simulink model "Hybrid_final_project_computer"  (R2022a)
settings: Solver=FixedStepAuto  StartTime=0.0  StopTime=25.0  RelTol=1e-3
model workspace (MAT data in the model file):
  Constant_a = Simulink.Parameter
  Constant_a.Value = [0  0.3  0.4  0.3; 0.3  0  0.5  0; 0.4  0.5  0  0.3; 0.3  0  0.3  0]
  Constant_a.DataType = 'auto'
  Constant_a.Complexity = 'real'
  Constant_a.Dimensions = [4 4]
  Constant_b = Simulink.Parameter
  Constant_b.Value = [0.3; 0.2; 0.5; 0.4]
  Constant_b.DataType = 'auto'
  Constant_b.Complexity = 'real'
  Constant_b.Dimensions = [4 1]
  Initial_Room_Temps = Simulink.Parameter
  Initial_Room_Temps.Value = [16.5; 16.5; 16.5; 16.5]
  Initial_Room_Temps.DataType = 'auto'
  Initial_Room_Temps.Complexity = 'real'
  Initial_Room_Temps.Dimensions = [4 1]
  constant_c = Simulink.Parameter
  constant_c.Value = [9; 7; 11; 7]
  constant_c.DataType = 'auto'
  constant_c.Complexity = 'real'
  constant_c.Dimensions = [4 1]
  dif_temps = Simulink.Parameter
  dif_temps.Value = [1; 1; 1; 1]
  dif_temps.DataType = 'auto'
  dif_temps.Complexity = 'real'
  dif_temps.Dimensions = [4 1]
  get_temps = Simulink.Parameter
  get_temps.Value = [17; 16; 16; 17]
  get_temps.DataType = 'auto'
  get_temps.Complexity = 'real'
  get_temps.Dimensions = [4 1]
  initial_placement = Simulink.Parameter
  initial_placement.Value = [0; 1; 1; 0]
  initial_placement.DataType = 'auto'
  initial_placement.Complexity = 'real'
  initial_placement.Dimensions = [4 1]
  off_temps = Simulink.Parameter
  off_temps.Value = [20; 20; 20; 20]
  off_temps.DataType = 'auto'
  off_temps.Complexity = 'real'
  off_temps.Dimensions = [4 1]
  on_temps = Simulink.Parameter
  on_temps.Value = [19; 19; 19; 19]
  on_temps.DataType = 'auto'
  on_temps.Complexity = 'real'
  on_temps.Dimensions = [4 1]
settings Model: Creator=jamieshatsky  LastModifiedBy=jamieshatsky
settings DebuggingCC: UnderSpecifiedDimensionMsg=warning

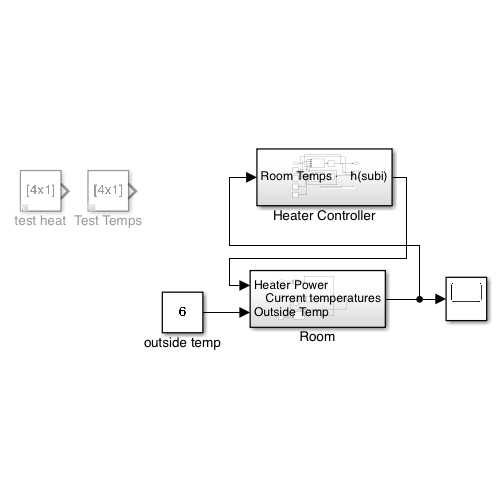
[thumbnail: Simulink's stored preview of the top-level diagram]
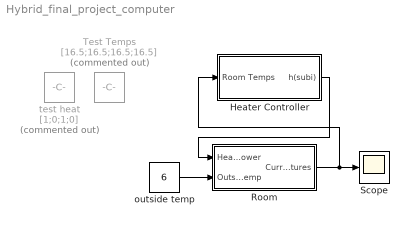
== system Hybrid_final_project_computer ==
  Heater Controller : Subsystem
  Room : Subsystem
  Scope : Scope
  Test Temps : Constant  Commented=on  Value=[16.5;16.5;16.5;16.5]
  outside temp : Constant  Value=6
  test heat : Constant  Commented=on  Value=[1;0;1;0]
  wires:
  outside temp/1 -> Room/2(Outside Temp)
  Room/1(Current temperatures) -> Heater Controller/1(Room Temps), Scope/1
  Heater Controller/1(h(subi)) -> Room/1(Heater Power)

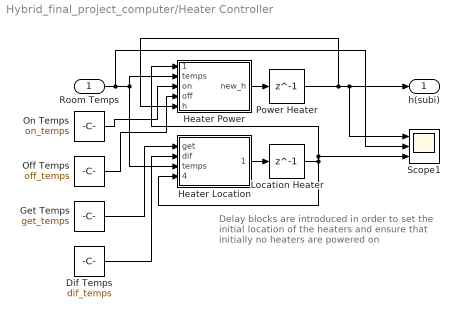
== system Hybrid_final_project_computer/Heater Controller ==
  note: Delay blocks are introduced in order to set the initial location of the heaters
      | and ensure that initially no heaters are powered on
  Room Temps : Inport
  Dif Temps : Constant  Value=dif_temps
  Get Temps : Constant  Value=get_temps
  Heater Location : MATLAB Function  TreatAsAtomicUnit=on
  Heater Power : MATLAB Function  TreatAsAtomicUnit=on
  Location Heater : Delay  DelayLength=1  InitialCondition=initial_placement
  Off Temps : Constant  Value=off_temps
  On Temps : Constant  Value=on_temps
  Power Heater : Delay  DelayLength=1  InitialCondition=[0;0;0;0]
  Scope1 : Scope  NumInputPorts=3
  h(subi) : Outport
  wires:
  Heater Location/1(new_location) -> Location Heater/1
  Room Temps/1 -> Scope1/2, Heater Location/3(temps), Heater Power/2(temps)
  Location Heater/1 -> Heater Power/1(location), Scope1/3, Heater Location/4(location)
  On Temps/1 -> Heater Power/3(on)
  Off Temps/1 -> Heater Power/4(off)
  Get Temps/1 -> Heater Location/1(get)
  Dif Temps/1 -> Heater Location/2(dif)
  Heater Power/1(new_h) -> Power Heater/1
  Power Heater/1 -> Scope1/1, h(subi)/1, Heater Power/5(h)

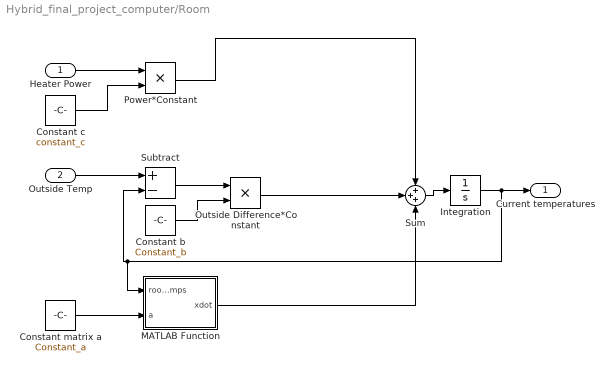
== system Hybrid_final_project_computer/Room ==
  Heater Power : Inport  PortDimensions=4
  Outside Temp : Inport  Port=2
  Constant b : Constant  Value=Constant_b
  Constant c : Constant  Value=constant_c
  Constant matrix a : Constant  Value=Constant_a  VectorParams1D=off
  Integration : Integrator  InitialCondition=Initial_Room_Temps
  MATLAB Function : MATLAB Function  TreatAsAtomicUnit=on
  Outside Difference*Constant : Product
  Power*Constant : Product
  Subtract : Sum  Inputs=+-
  Sum : Sum  Inputs=+++
  Current temperatures : Outport
  wires:
  Heater Power/1 -> Power*Constant/1
  Constant c/1 -> Power*Constant/2
  Power*Constant/1 -> Sum/1
  Outside Temp/1 -> Subtract/1
  Subtract/1 -> Outside Difference*Constant/1
  Constant b/1 -> Outside Difference*Constant/2
  Outside Difference*Constant/1 -> Sum/2
  Constant matrix a/1 -> MATLAB Function/2(a)
  Sum/1 -> Integration/1
  Integration/1 -> Subtract/2, MATLAB Function/1(room_temps), Current temperatures/1
  MATLAB Function/1(xdot) -> Sum/3

== matlab function Hybrid_final_project_computer/Heater Controller/Heater Location ==
  data: new_location output; get input; dif input; temps input; location input
function new_location = fcn(get, dif, temps, location)
    for i = 1:numel(temps)
        if location(i) == 0 % Only look to move heater if a room doesn't have one
            for j = 1:numel(temps)
                % Swap location of heater if room i does not  have a heater,
                % room j has a heater, the temperature in room i is less
                % than or equal to get, and the difference in temperatures 
                % between room j and room i is greater than or equal to dif
                if location(j) == 1 && temps(i) <= get(i) && temps(j) - temps(i) >= dif(i)
                    location(j) = 0; % Swap locations of heaters
                    location(i) = 1;
                    % We will swap heaters with the first room that 
                    % meets the requirements and then break out of
                    % the loop
                    break 
                end 
            end
        end
    end

    new_location = location;
end

== matlab function Hybrid_final_project_computer/Room/MATLAB Function ==
  data: room_temps input; xdot output; a input
function xdot  = fcn(room_temps, a)
    sum = 0;
    for j = 1:numel(room_temps)
        if j ~= 1
            sum = ((room_temps(j) - room_temps(1)) * a(1, j)) + sum;
        end
    end
    xdot1 = sum;

    sum = 0;
    for j = 1:numel(room_temps)
        if j ~= 2
            sum = ((room_temps(j) - room_temps(2)) * a(2, j)) + sum;
        end
    end
    xdot2 = sum;

    sum = 0;
    for j = 1:numel(room_temps)
        if j ~= 3
            sum = ((room_temps(j) - room_temps(3)) * a(3, j)) + sum;
        end
    end
    xdot3 = sum;

    sum = 0;
    for j = 1:numel(room_temps)
        if j ~= 4
            sum = ((room_temps(j) - room_temps(4)) * a(4, j)) + sum;
        end
    end
    xdot4 = sum;

    xdot = [xdot1;xdot2;xdot3;xdot4];
end

== matlab function Hybrid_final_project_computer/Heater Controller/Heater Power ==
  data: location input; new_h output; temps input; on input; off input; h input
% The parameter h represents the heater power array of the previous time
% step and the return value of the function is the heater power array of
% the current time step
function new_h = fcn(location, temps, on, off, h) 
    % Only turn heater on or off if the room has a heater
    if location(1) == 1
        if temps(1) <= on(1)
            h(1) = 1; % Turn heater on
        elseif temps(1) >= off(1)
            h(1) = 0; % Turn heater off
        end
    else
        % If this room doesn't have a heater, it is impossible for the
        % heater to be on in the room 
        h(1) = 0;
    end

    if location(2) == 1
        if temps(2) <= on(2)
            h(2) = 1; % Turn heater on
        elseif temps(2) >= off(2)
            h(2) = 0; % Turn heater off
        end
    else
        % If this room doesn't have a heater, it is impossible for the
        % heater to be on in the room 
        h(2) = 0;
    end

    if location(3) == 1
        if temps(3) <= on(3)
            h(3) = 1; % Turn heater on
        elseif temps(3) >= off(3)
            h(3) = 0; % Turn heater off
        end
    else
        % If this room doesn't have a heater, it is impossible for the
        % heater to be on in the room 
        h(3) = 0;
    end

    if location(4) == 1
        if temps(4) <= on(4)
            h(4) = 1; % Turn heater on
        elseif temps(4) >= off(4)
            h(4) = 0; % Turn heater off
        end
    else
        % If this room doesn't have a heater, it is impossible for the
        % heater to be on in the room 
        h(4) = 0;
    end

    new_h = h;
end
